simulink model "Controller"  (R2022a)
settings: Solver=VariableStepAuto  StartTime=0.0  StopTime=5  RelTol=1e-3
values from neighbouring files (symbols this model uses):
  count_rate = 1/f    (= 0.0399361022364)    [ControllerModel.m]
  f = 25.04    [ControllerModel.m]
  Kd = 0    [ControllerModel.m]
  Ki = 0    [ControllerModel.m]
  Km = 4.44*10^-3    (= 0.00444)    [ControllerModel.m]
  Kp = 1    [ControllerModel.m]
  L = 0.026*10^-3    (= 2.6e-05)    [ControllerModel.m]
  R = 0.43    [ControllerModel.m]
libraries: simulink_extras x5, cstblocks x1
settings Model: Creator=francesfarmer  LastModifiedBy=overt
settings SolverCC: AlgebraicLoopSolver=TrustRegion
settings DebuggingCC: UnconnectedInputMsg=warning  UnconnectedOutputMsg=warning  UnconnectedLineMsg=warning  SFMachineParentedDataDiag=warning
settings RTWCC: DLArmComputeVersion=19.05

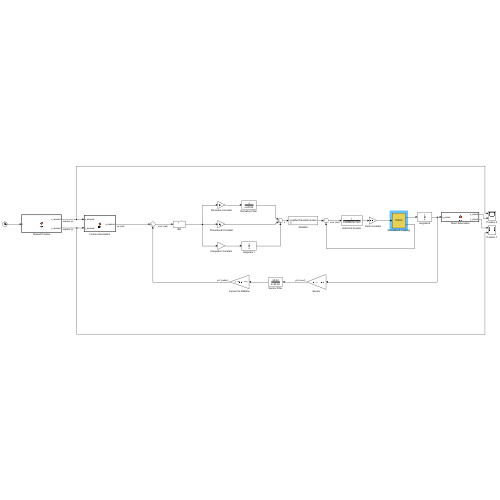
[thumbnail: Simulink's stored preview of the top-level diagram]
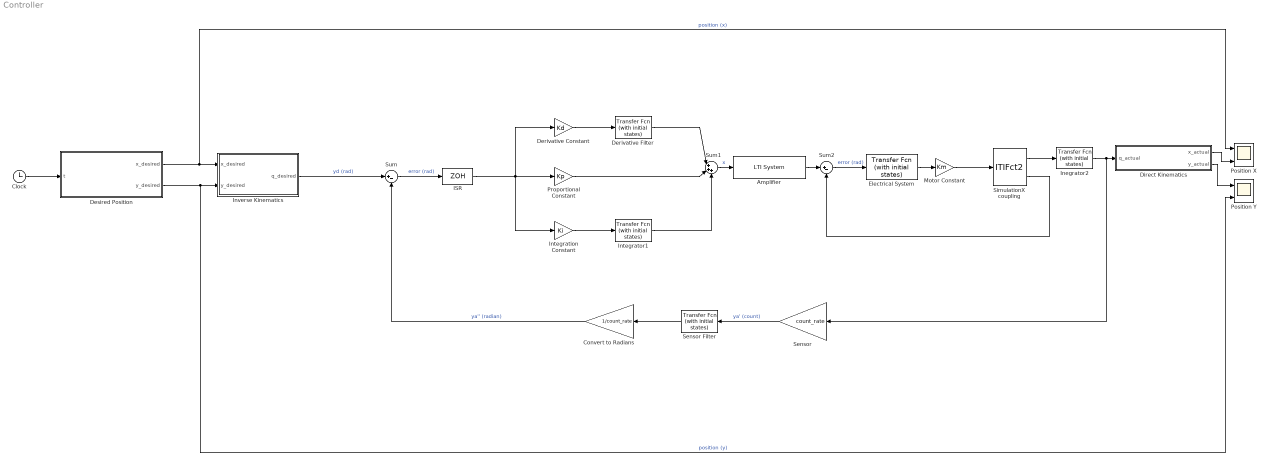
== system Controller ==
  Amplifier : cstblocks/LTI System  sys=AmplifierTransferFunction  IC=[]
  Clock : Clock
  Convert to Radians : Gain  Gain=1/count_rate
  Derivative Constant : Gain  Gain=Kd
  "Derivative Filter " : simulink_extras/Additional Linear/Transfer Fcn (with initial states)  N=[1 0]  D="[1  f]"  X0=0
  Desired Position : MATLAB Function  TreatAsAtomicUnit=on
  Direct Kinematics : MATLAB Function  TreatAsAtomicUnit=on
  Electrical System : simulink_extras/Additional Linear/Transfer Fcn (with initial states)  N=[1]  D="[L  R]"  X0=0
  ISR : ZeroOrderHold  SampleTime=1/f
  Inegrator2 : simulink_extras/Additional Linear/Transfer Fcn (with initial states)  N=[1]  D="[1  0]"  X0=0
  Integration Constant : Gain  Gain=Ki
  Integrator1 : simulink_extras/Additional Linear/Transfer Fcn (with initial states)  N=[1]  D="[1  0]"  X0=0
  Inverse Kinematics : MATLAB Function  TreatAsAtomicUnit=on
  Motor Constant : Gain  Gain=Km
  Position X : Scope  NumInputPorts=2
  Position Y : Scope  NumInputPorts=2
  Proportional Constant : Gain  Gain=Kp
  Sensor : Gain  Gain=count_rate
  Sensor Filter : simulink_extras/Additional Linear/Transfer Fcn (with initial states)  N=[f]  D=[1 f]  X0=0
  SimulationX coupling : S-Function  FunctionName=ITIFct2  Parameters=ip, port, ts, nIn, nOut  SFunctionDeploymentMode=off  EnableBusSupport=off  mask{ip='localhost', port=4097, ts=0.001, nIn=1, nOut=2}
      mask prompts: ip "Address: ip"; port "Port Number: port [-]"; ts "Communication Step Size: ts [s]"; nIn "Input Vector Dimension (to SimulationX): nIn [-]"; nOut "Output Vector Dimension (from SimulationX): nOut [-]"
      mask help: Coupling Element
  Sum : Sum  Inputs=|+-
  Sum1 : Sum  Inputs=|+++
  Sum2 : Sum  Inputs=|+-
  wires:
  Desired Position/1(x_desired) -> Inverse Kinematics/1(x_desired), Position X/1  "position (x)"
  Desired Position/2(y_desired) -> Position Y/2, Inverse Kinematics/2(y_desired)  "position (y)"
  Sum/1 -> ISR/1  "error (rad)"
  Integration Constant/1 -> Integrator1/1
  Proportional Constant/1 -> Sum1/2
  Integrator1/1 -> Sum1/3
  Derivative Constant/1 -> "Derivative Filter "/1
  Sum1/1 -> Amplifier/1  "x"
  Inverse Kinematics/1(q_desired) -> Sum/1  "yd (rad)"
  "Derivative Filter "/1 -> Sum1/1
  Clock/1 -> Desired Position/1(t)
  Electrical System/1 -> Motor Constant/1
  ISR/1 -> Derivative Constant/1, Proportional Constant/1, Integration Constant/1
  Sensor Filter/1 -> Convert to Radians/1
  Convert to Radians/1 -> Sum/2  "ya'' (radian)"
  Sensor/1 -> Sensor Filter/1  "ya' (count)"
  Direct Kinematics/2(y_actual) -> Position Y/1
  Direct Kinematics/1(x_actual) -> Position X/2
  Inegrator2/1 -> Sensor/1, Direct Kinematics/1(q_actual)
  SimulationX coupling/1 -> Inegrator2/1
  Motor Constant/1 -> SimulationX coupling/1
  Amplifier/1 -> Sum2/1
  Sum2/1 -> Electrical System/1  "error (rad)"
  SimulationX coupling/2 -> Sum2/2

== matlab function Controller/Desired Position ==
  data: t input; x_desired output; y_desired output
function [x_desired,y_desired] = fcn(t) %This function is used to determine the path of the arm //ba

y_desired =(98.88*10^-3)*sin(t);
x_desired=(98.88*10^-3)*cos(t);

== matlab function Controller/Direct Kinematics ==
  data: x_actual output; y_actual output; q_actual input
function [x_actual, y_actual]  = fcn(q_actual)

y_actual = (98.88*10^-3)*sin(q_actual); %multiply by the distance from joint1 to joint 2
x_actual=(98.88*10^-3)*cos(q_actual); %multiply by the distance from joint1 to joint2

== matlab function Controller/Inverse Kinematics ==
  data: x_desired input; q_desired output; y_desired input
function q_desired = fcn(x_desired,y_desired) %Inverse Kinematics
q_desired = atan(y_desired/x_desired);
